simulink model "RajamaniController"  (R2018a)
settings: Solver=ode45  StartTime=0.0  StopTime=inf  FixedStep=0.002  RelTol=1e-3  EnableMultiTasking=on
values from neighbouring files (symbols this model uses):
  alpha_f0 = states(7)    [IS_2impulse.m]    (also in IS_3impulse.m; IS_4impulse.m; InputShaper.m; InputShaper2.m = 0)
  alpha_r0 = states(8)    [IS_2impulse.m]    (also in IS_3impulse.m; IS_4impulse.m; InputShaper.m; InputShaper2.m = 0)
  Bx_ash_f = 11.7    [ISData.m]    (also in SbWdata.m; pacjeka_params.m)
  Bx_ash_r = 11.1    [ISData.m]    (also in SbWdata.m; pacjeka_params.m)
  Bx_snow_f = 10.2    [ISData.m]    (also in SbWdata.m; pacjeka_params.m)
  Bx_snow_r = 9.71    [ISData.m]    (also in SbWdata.m; pacjeka_params.m)
  Bx_wash_f = 12    [ISData.m]    (also in SbWdata.m; pacjeka_params.m)
  Bx_wash_r = 11.5    [ISData.m]    (also in SbWdata.m; pacjeka_params.m)
  By_ash_f = 8.86    [ISData.m]    (also in SbWdata.m; pacjeka_params.m)
  By_ash_r = 9.30    (= 9.3)    [ISData.m]    (also in SbWdata.m; pacjeka_params.m)
  By_snow_f = 19.1    [ISData.m]    (also in SbWdata.m; pacjeka_params.m)
  By_snow_r = 20.0    (= 20)    [ISData.m]    (also in SbWdata.m; pacjeka_params.m)
  By_wash_f = 10.7    [ISData.m]    (also in SbWdata.m; pacjeka_params.m)
  By_wash_r = 11.3    [ISData.m]    (also in SbWdata.m; pacjeka_params.m)
  C_alpha_f = 1830*0.45*0.165*57.29578    (= 7785.20734695)    [IS_2impulse.m]    (also in IS_3impulse.m; IS_4impulse.m; InputShaper.m = 8650.2303855; InputShaper2.m = 8650.2303855)
  C_alpha_r = 1830*0.55*0.165*57.29578    (= 9515.25342405)    [IS_2impulse.m]    (also in IS_3impulse.m; IS_4impulse.m; InputShaper.m = 8650.2303855; InputShaper2.m = 8650.2303855)
  Cx_ash_f = 1.69    [ISData.m]    (also in SbWdata.m; pacjeka_params.m)
  Cx_ash_r = 1.69    [ISData.m]    (also in SbWdata.m; pacjeka_params.m)
  Cx_snow_f = 1.96    [ISData.m]    (also in SbWdata.m; pacjeka_params.m)
  Cx_snow_r = 1.96    [ISData.m]    (also in SbWdata.m; pacjeka_params.m)
  Cx_wash_f = 1.80    (= 1.8)    [ISData.m]    (also in SbWdata.m; pacjeka_params.m)
  Cx_wash_r = 1.80    (= 1.8)    [ISData.m]    (also in SbWdata.m; pacjeka_params.m)
  Cy_ash_f = 1.19    [ISData.m]    (also in SbWdata.m; pacjeka_params.m)
  Cy_ash_r = 1.19    [ISData.m]    (also in SbWdata.m; pacjeka_params.m)
  Cy_snow_f = 0.550    (= 0.55)    [ISData.m]    (also in SbWdata.m; pacjeka_params.m)
  Cy_snow_r = 0.550    (= 0.55)    [ISData.m]    (also in SbWdata.m; pacjeka_params.m)
  Cy_wash_f = 1.07    [ISData.m]    (also in SbWdata.m; pacjeka_params.m)
  Cy_wash_r = 1.07    [ISData.m]    (also in SbWdata.m; pacjeka_params.m)
  D_phi = 16000    [ISData.m]    (also in IS_2impulse.m; IS_3impulse.m; IS_4impulse.m; InputShaper.m)
  D_theta = 30960    [ISData.m]    (also in IS_2impulse.m; IS_3impulse.m; IS_4impulse.m; InputShaper.m)
  delta_r = 0    [ISData.m]    (also in IS_2impulse.m; IS_3impulse.m; IS_4impulse.m; InputShaper.m)
  epsilon = 0.4    [ISData.m]    (also in IS_2impulse.m; IS_3impulse.m; IS_4impulse.m; InputShaper.m)
  Ex_ash_f = 0.377    [ISData.m]    (also in SbWdata.m; pacjeka_params.m)
  Ex_ash_r = 0.362    [ISData.m]    (also in SbWdata.m; pacjeka_params.m)
  Ex_snow_f = 0.651    [ISData.m]    (also in SbWdata.m; pacjeka_params.m)
  Ex_snow_r = 0.624    [ISData.m]    (also in SbWdata.m; pacjeka_params.m)
  Ex_wash_f = 0.313    [ISData.m]    (also in SbWdata.m; pacjeka_params.m)
  Ex_wash_r = 0.300    (= 0.3)    [ISData.m]    (also in SbWdata.m; pacjeka_params.m)
  Ey_ash_f = -1.21    [ISData.m]    (also in SbWdata.m; pacjeka_params.m)
  Ey_ash_r = -1.11    [ISData.m]    (also in SbWdata.m; pacjeka_params.m)
  Ey_snow_f = -2.1    [ISData.m]    (also in SbWdata.m; pacjeka_params.m)
  Ey_snow_r = -1.93    [ISData.m]    (also in SbWdata.m; pacjeka_params.m)
  Ey_wash_f = -2.14    [ISData.m]    (also in SbWdata.m; pacjeka_params.m)
  Ey_wash_r = -1.97    [ISData.m]    (also in SbWdata.m; pacjeka_params.m)
  g = 9.81    [ISData.m]    (also in IS_2impulse.m; IS_3impulse.m; IS_4impulse.m; InputShaper.m)
  h = 0.5    [ISData.m]    (also in IS_2impulse.m; IS_3impulse.m; IS_4impulse.m; InputShaper.m)
  Iw = 4    [ISData.m]    (also in IS_2impulse.m; IS_3impulse.m; IS_4impulse.m; InputShaper.m)
  Ixx = 602.1923    [ISData.m]    (also in IS_2impulse.m; IS_3impulse.m; IS_4impulse.m; InputShaper.m)
  Iyy = 2.7370e+03    (= 2737)    [ISData.m]    (also in IS_2impulse.m; IS_3impulse.m; IS_4impulse.m; InputShaper.m)
  Iz = Izz    (= 3070)    [IS_2impulse.m]    (also in IS_3impulse.m; IS_4impulse.m; InputShaper.m; InputShaper2.m)
  Izz = 3070    [ISData.m]    (also in IS_2impulse.m; IS_3impulse.m; IS_4impulse.m; InputShaper.m)
  K_phi = 178000    [ISData.m]    (also in IS_2impulse.m; IS_3impulse.m; IS_4impulse.m; InputShaper.m)
  K_theta = 363540    [ISData.m]    (also in IS_2impulse.m; IS_3impulse.m; IS_4impulse.m; InputShaper.m)
  Ksbw = 1    [SbWdata.m]
  l = l_f+l_r    (= 2.67)    [IS_2impulse.m]    (also in IS_3impulse.m; IS_4impulse.m; InputShaper.m; InputShaper2.m)
  l_f = 1.2110    (= 1.211)    [ISData.m]    (also in IS_2impulse.m; IS_3impulse.m; IS_4impulse.m; InputShaper.m)
  l_p = Iz/(m*l_r)    (= 1.14982565347)    [IS_2impulse.m]    (also in IS_3impulse.m; IS_4impulse.m; InputShaper.m; InputShaper2.m)
  l_r = 1.4590    (= 1.459)    [ISData.m]    (also in IS_2impulse.m; IS_3impulse.m; IS_4impulse.m; InputShaper.m)
  m = 1830    [ISData.m]    (also in IS_2impulse.m; IS_3impulse.m; IS_4impulse.m; InputShaper.m)
  mu_x_ash_f = 1.20    (= 1.2)    [ISData.m]    (also in SbWdata.m; pacjeka_params.m)
  mu_x_ash_r = 1.20    (= 1.2)    [ISData.m]    (also in SbWdata.m; pacjeka_params.m)
  mu_x_snow_f = 0.407    [ISData.m]    (also in SbWdata.m; pacjeka_params.m)
  mu_x_snow_r = 0.409    [ISData.m]    (also in SbWdata.m; pacjeka_params.m)
  mu_x_wash_f = 1.06    [ISData.m]    (also in SbWdata.m; pacjeka_params.m)
  mu_x_wash_r = 1.07    [ISData.m]    (also in SbWdata.m; pacjeka_params.m)
  mu_y_ash_f = 0.935    [ISData.m]    (also in SbWdata.m; pacjeka_params.m)
  mu_y_ash_r = 0.961    [ISData.m]    (also in SbWdata.m; pacjeka_params.m)
  mu_y_snow_f = 0.383    [ISData.m]    (also in SbWdata.m; pacjeka_params.m)
  mu_y_snow_r = 0.394    [ISData.m]    (also in SbWdata.m; pacjeka_params.m)
  mu_y_wash_f = 0.885    [ISData.m]    (also in SbWdata.m; pacjeka_params.m)
  mu_y_wash_r = 0.911    [ISData.m]    (also in SbWdata.m; pacjeka_params.m)
  omega0 = Vx0/Rw    (= 64.7813411079)    [ISData.m]    (also in IS_2impulse.m = 74.1; IS_3impulse.m = 74.1; IS_4impulse.m = 74.1; InputShaper.m = 55.5666666667)
  omega_f0 = states(5)    [IS_2impulse.m]    (also in IS_3impulse.m; IS_4impulse.m; InputShaper.m; InputShaper2.m = 55.5666666667)
  omega_r0 = states(6)    [IS_2impulse.m]    (also in IS_3impulse.m; IS_4impulse.m; InputShaper.m; InputShaper2.m = 55.5666666667)
  psi0 = states(2)    [IS_2impulse.m]    (also in IS_3impulse.m; IS_4impulse.m; InputShaper.m; InputShaper2.m = 0)
  psi_dot0 = states(1)    [IS_2impulse.m]    (also in IS_3impulse.m; IS_4impulse.m; InputShaper.m; InputShaper2.m = 0)
  Px0 = states(9)    [IS_2impulse.m]    (also in IS_3impulse.m; IS_4impulse.m; InputShaper.m; InputShaper2.m = 0)
  Py0 = states(10)    [IS_2impulse.m]    (also in IS_3impulse.m; IS_4impulse.m; InputShaper.m; InputShaper2.m = 0)
  Re = Rw    (= 0.3)    [IS_2impulse.m]    (also in IS_3impulse.m; IS_4impulse.m; InputShaper.m; InputShaper2.m)
  road = 1    [ISData.m]    (also in IS_2impulse.m; IS_3impulse.m; IS_4impulse.m; InputShaper.m)
  Rw = 0.3430    (= 0.343)    [ISData.m]    (also in IS_2impulse.m = 0.3; IS_3impulse.m = 0.3; IS_4impulse.m = 0.3; InputShaper.m = 0.3)
  sigma = epsilon    (= 0.4)    [IS_2impulse.m]    (also in IS_3impulse.m; IS_4impulse.m; InputShaper.m; InputShaper2.m)
  Ts = 0.001    [ISData.m]    (also in IS_2impulse.m; IS_3impulse.m; IS_4impulse.m; InputShaper.m)
  Tsmall = 0.001    [ISData.m]    (also in IS_2impulse.m; IS_3impulse.m; IS_4impulse.m; InputShaper.m)
  Vx0 = 22.22    [ISData.m]    (also in IS_2impulse.m = states(3); IS_3impulse.m = states(3); IS_4impulse.m = states(3); InputShaper.m = states(3))
  Vy0 = states(4)    [IS_2impulse.m]    (also in IS_3impulse.m; IS_4impulse.m; InputShaper.m; InputShaper2.m = 0)
  w = 0.7700    (= 0.77)    [ISData.m]    (also in IS_2impulse.m; IS_3impulse.m; IS_4impulse.m; InputShaper.m)
(part 3 of 3)

== system RajamaniController/Vehicle_Sim/Vehicle_model/phi_subsystem/phi_ddot_numerator_subsystem ==
  FY : Inport  OutDataTypeStr=double  SampleTime=Ts
  psi_dot : Inport  Port=2  OutDataTypeStr=double  SampleTime=Tsmall
  phi_dot : Inport  Port=3  OutDataTypeStr=double  SampleTime=Tsmall
  phi : Inport  Port=4  OutDataTypeStr=double  SampleTime=Tsmall
  theta_dot : Inport  Port=5  OutDataTypeStr=double  SampleTime=Tsmall
  theta : Inport  Port=6  OutDataTypeStr=double  SampleTime=Tsmall
  Iyy : Inport  Port=7  OutDataTypeStr=double  SampleTime=Ts
  Izz : Inport  Port=8  OutDataTypeStr=double  SampleTime=Ts
  K_phi : Inport  Port=9  OutDataTypeStr=double  SampleTime=Ts
  D_phi : Inport  Port=10  OutDataTypeStr=double  SampleTime=Ts
  h : Inport  Port=11  OutDataTypeStr=double  SampleTime=Ts
  Add : Sum
  Add1 : Sum  Inputs=+++
  Add2 : Sum
  Add3 : Sum  Inputs=+-
  Add4 : Sum
  Add7 : Sum  Inputs=+++
  Divide{,1..4,7..12} (11 alike) : Product  Inputs=**
  Divide5 : Product  Inputs=****
  Divide6 : Product  Inputs=****
  Gain : Gain  Gain=m*g
  Gain2 : Gain  Gain=-1
  Gain3 : Gain  Gain=-1
  Square : Math  Operator=square  RndMeth=Zero  SaturateOnIntegerOverflow=on
  Square1 : Math  Operator=square  RndMeth=Zero  SaturateOnIntegerOverflow=on
  Trigonometric Function : Trigonometry
  Trigonometric Function1 : Trigonometry  Operator=cos
  Trigonometric Function2 : Trigonometry  Operator=cos
  Trigonometric Function3 : Trigonometry
  phi_ddot_numerator : Outport  OutDataTypeStr=double  SampleTime=Tsmall
  wires:
  phi_dot/1 -> Divide1/1, Divide6/3  "phi_dot"
  psi_dot/1 -> Divide4/1, Divide5/4, Divide11/2  "psi_dot"
  Divide6/1 -> Add4/2
  phi/1 -> Divide/1, Trigonometric Function/1, Trigonometric Function1/1  "phi"
  theta/1 -> Trigonometric Function2/1, Trigonometric Function3/1  "theta"
  FY/1 -> Divide2/1  "FY"
  theta_dot/1 -> Divide11/1  "theta_dot"
  Gain2/1 -> Divide/2
  Gain3/1 -> Divide1/2
  Divide1/1 -> Add1/2
  Divide9/1 -> Add2/2
  Divide12/1 -> Add1/3
  Add/1 -> Divide12/1
  Divide3/1 -> Add/2
  Add2/1 -> Divide10/1
  Iyy/1 -> Divide9/2, Add3/1  "Iyy"
  Divide2/1 -> Divide3/1
  Square1/1 -> Divide8/2
  Izz/1 -> Add3/2, Divide8/1  "Izz"
  Add3/1 -> Divide4/2  "del_Iyz"
  Gain/1 -> Add/1
  Add7/1 -> phi_ddot_numerator/1
  Divide8/1 -> Add2/1
  Divide4/1 -> Divide7/1
  Add4/1 -> Divide7/2
  Trigonometric Function2/1 -> Divide3/2, Divide5/3  "cosTheta"
  Divide11/1 -> Divide10/2
  Divide5/1 -> Add4/1
  Divide7/1 -> Add7/2
  Square/1 -> Divide9/1
  Trigonometric Function1/1 -> Divide2/2, Divide5/2, Square/1, Divide6/2  "cosPhi"
  Divide10/1 -> Add7/3
  Add1/1 -> Add7/1
  Trigonometric Function3/1 -> Divide6/4  "sinTheta"
  Divide/1 -> Add1/1
  Trigonometric Function/1 -> Divide5/1, Divide6/1, Square1/1, Gain/1  "sinPhi"
  K_phi/1 -> Gain2/1  "K_phi"
  D_phi/1 -> Gain3/1  "D_phi"
  h/1 -> Divide12/2  "h"

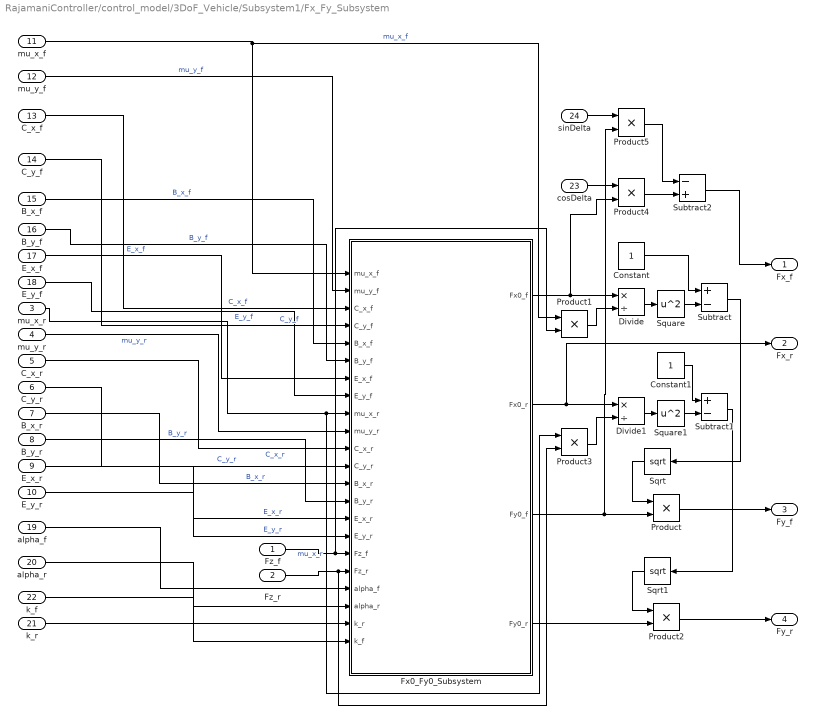
== system RajamaniController/control_model/3DoF_Vehicle/Subsystem1/Fx_Fy_Subsystem ==
  Fz_f : Inport
  Fz_r : Inport  Port=2
  mu_x_r : Inport  Port=3
  mu_y_r : Inport  Port=4
  C_x_r : Inport  Port=5
  C_y_r : Inport  Port=6
  B_x_r : Inport  Port=7
  B_y_r : Inport  Port=8
  E_x_r : Inport  Port=9
  E_y_r : Inport  Port=10
  mu_x_f : Inport  Port=11
  mu_y_f : Inport  Port=12
  C_x_f : Inport  Port=13
  C_y_f : Inport  Port=14
  B_x_f : Inport  Port=15
  B_y_f : Inport  Port=16
  E_x_f : Inport  Port=17
  E_y_f : Inport  Port=18
  alpha_f : Inport  Port=19
  alpha_r : Inport  Port=20
  k_r : Inport  Port=21
  k_f : Inport  Port=22
  cosDelta : Inport  Port=23
  sinDelta : Inport  Port=24
  Constant : Constant
  Constant1 : Constant
  Divide : Product  Inputs=*/
  Divide1 : Product  Inputs=*/
  Fx0_Fy0_Subsystem : Subsystem
  Product{,1..5} (6 alike) : Product
  Sqrt : Sqrt  SaturateOnIntegerOverflow=on
  Sqrt1 : Sqrt  SaturateOnIntegerOverflow=on
  Square : Math  Operator=square  SaturateOnIntegerOverflow=on
  Square1 : Math  Operator=square  SaturateOnIntegerOverflow=on
  Subtract : Sum  Inputs=+-
  Subtract1 : Sum  Inputs=+-
  Subtract2 : Sum  Inputs=-+
  Fx_f : Outport
  Fx_r : Outport  Port=2
  Fy_f : Outport  Port=3
  Fy_r : Outport  Port=4
  wires:
  B_x_r/1 -> Fx0_Fy0_Subsystem/13(B_x_r)  "B_x_r"
  mu_y_r/1 -> Fx0_Fy0_Subsystem/10(mu_y_r)  "mu_y_r"
  C_x_r/1 -> Fx0_Fy0_Subsystem/11(C_x_r)  "C_x_r"
  E_y_r/1 -> Fx0_Fy0_Subsystem/16(E_y_r)  "E_y_r"
  mu_x_r/1 -> Fx0_Fy0_Subsystem/9(mu_x_r), Product3/1  "mu_x_r"
  C_y_r/1 -> Fx0_Fy0_Subsystem/12(C_y_r)  "C_y_r"
  E_x_r/1 -> Fx0_Fy0_Subsystem/15(E_x_r)  "E_x_r"
  B_y_r/1 -> Fx0_Fy0_Subsystem/14(B_y_r)  "B_y_r"
  B_x_f/1 -> Fx0_Fy0_Subsystem/5(B_x_f)  "B_x_f"
  mu_y_f/1 -> Fx0_Fy0_Subsystem/2(mu_y_f)  "mu_y_f"
  C_x_f/1 -> Fx0_Fy0_Subsystem/3(C_x_f)  "C_x_f"
  E_y_f/1 -> Fx0_Fy0_Subsystem/8(E_y_f)  "E_y_f"
  mu_x_f/1 -> Product1/1, Fx0_Fy0_Subsystem/1(mu_x_f)  "mu_x_f"
  C_y_f/1 -> Fx0_Fy0_Subsystem/4(C_y_f)  "C_y_f"
  E_x_f/1 -> Fx0_Fy0_Subsystem/7(E_x_f)  "E_x_f"
  B_y_f/1 -> Fx0_Fy0_Subsystem/6(B_y_f)  "B_y_f"
  Fz_f/1 -> Product1/2, Fx0_Fy0_Subsystem/17(Fz_f)
  Fz_r/1 -> Product3/2, Fx0_Fy0_Subsystem/18(Fz_r)
  alpha_f/1 -> Fx0_Fy0_Subsystem/19(alpha_f)
  alpha_r/1 -> Fx0_Fy0_Subsystem/20(alpha_r)
  k_f/1 -> Fx0_Fy0_Subsystem/22(k_f)
  k_r/1 -> Fx0_Fy0_Subsystem/21(k_r)
  Constant/1 -> Subtract/1
  Fx0_Fy0_Subsystem/1(Fx0_f) -> Product4/2, Divide/1
  Product1/1 -> Divide/2
  Divide/1 -> Square/1
  Subtract/1 -> Sqrt/1
  Square/1 -> Subtract/2
  Sqrt/1 -> Product/1
  Product/1 -> Fy_f/1
  Product2/1 -> Fy_r/1
  Fx0_Fy0_Subsystem/4(Fy0_r) -> Product2/2
  Sqrt1/1 -> Product2/1
  Divide1/1 -> Square1/1
  Square1/1 -> Subtract1/2
  Product3/1 -> Divide1/2
  Fx0_Fy0_Subsystem/2(Fx0_r) -> Fx_r/1, Divide1/1
  Constant1/1 -> Subtract1/1
  Subtract1/1 -> Sqrt1/1
  cosDelta/1 -> Product4/1
  Product4/1 -> Subtract2/2
  sinDelta/1 -> Product5/1
  Fx0_Fy0_Subsystem/3(Fy0_f) -> Product5/2, Product/2
  Product5/1 -> Subtract2/1
  Subtract2/1 -> Fx_f/1

== system RajamaniController/control_model/3DoF_Vehicle/Subsystem1/Fz_Subsystem ==
  Constant : Constant  Value=(m*g*l_f)/l
  Constant1 : Constant  Value=(m*g*l_r)/l
  Fz_f : Outport
  Fz_r : Outport  Port=2
  wires:
  Constant/1 -> Fz_r/1
  Constant1/1 -> Fz_f/1

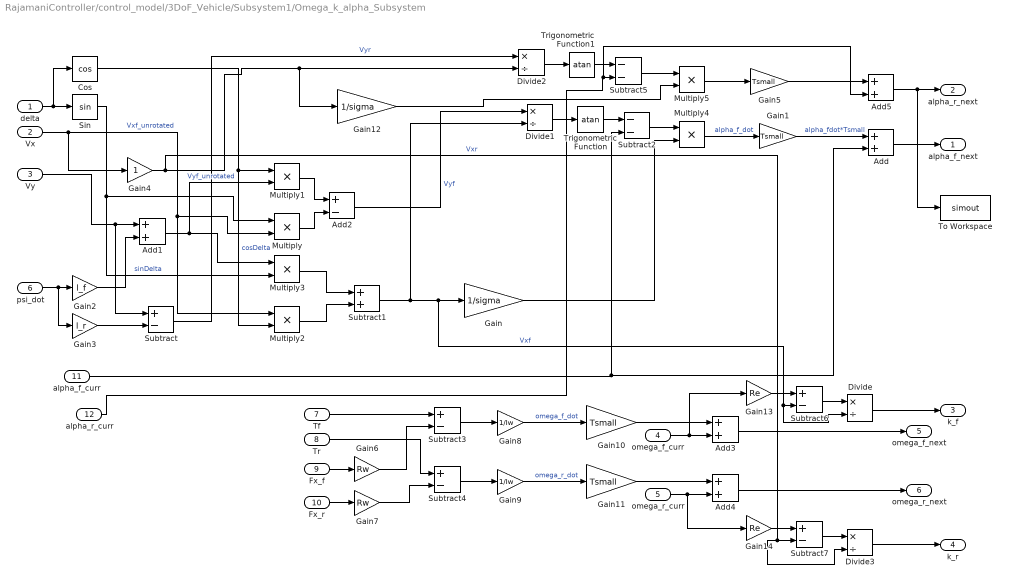
== system RajamaniController/control_model/3DoF_Vehicle/Subsystem1/Omega_k_alpha_Subsystem ==
  delta : Inport
  Vx : Inport  Port=2
  Vy : Inport  Port=3
  omega_f_curr : Inport  Port=4
  omega_r_curr : Inport  Port=5
  psi_dot : Inport  Port=6
  Tf : Inport  Port=7
  Tr : Inport  Port=8
  Fx_f : Inport  Port=9
  Fx_r : Inport  Port=10
  alpha_f_curr : Inport  Port=11
  alpha_r_curr : Inport  Port=12
  Add{,1,3..5} (5 alike) : Sum
  Add2 : Sum  Inputs=+-
  Cos : Trigonometry  Operator=cos
  Divide{,1..3} (4 alike) : Product  Inputs=*/
  Gain : Gain  Gain=1/sigma
  Gain{1,5,10..11} (4 alike) : Gain  Gain=Tsmall
  Gain12 : Gain  Gain=1/sigma
  Gain13 : Gain  Gain=Re
  Gain14 : Gain  Gain=Re
  Gain2 : Gain  Gain=l_f
  Gain3 : Gain  Gain=l_r
  Gain4 : Gain
  Gain6 : Gain  Gain=Rw
  Gain7 : Gain  Gain=Rw
  Gain8 : Gain  Gain=1/Iw
  Gain9 : Gain  Gain=1/Iw
  Multiply{,1..5} (6 alike) : Product
  Sin : Trigonometry
  Subtract{,3..4,6..7} (5 alike) : Sum  Inputs=+-
  Subtract1 : Sum
  Subtract2 : Sum  Inputs=--
  Subtract5 : Sum  Inputs=--
  To Workspace : ToWorkspace  VariableName=simout  SaveFormat=Timeseries  SampleTime=-1
  Trigonometric Function : Trigonometry  Operator=atan
  Trigonometric Function1 : Trigonometry  Operator=atan
  alpha_f_next : Outport
  alpha_r_next : Outport  Port=2
  k_f : Outport  Port=3
  k_r : Outport  Port=4
  omega_f_next : Outport  Port=5
  omega_r_next : Outport  Port=6
  wires:
  Fx_f/1 -> Gain6/1
  Fx_r/1 -> Gain7/1
  Tf/1 -> Subtract3/1
  Gain6/1 -> Subtract3/2
  Tr/1 -> Subtract4/1
  Gain7/1 -> Subtract4/2
  Subtract3/1 -> Gain8/1
  Subtract4/1 -> Gain9/1
  Gain8/1 -> Gain10/1  "omega_f_dot"
  Gain9/1 -> Gain11/1  "omega_r_dot"
  Gain10/1 -> Add3/1
  Gain11/1 -> Add4/1
  Add3/1 -> omega_f_next/1
  Add4/1 -> omega_r_next/1
  omega_f_curr/1 -> Gain13/1, Add3/2
  Multiply4/1 -> Gain1/1  "alpha_f_dot"
  Gain1/1 -> Add/1  "alpha_fdot*Tsmall"
  Divide1/1 -> Trigonometric Function/1
  omega_r_curr/1 -> Gain14/1, Add4/2
  psi_dot/1 -> Gain3/1, Gain2/1
  Gain2/1 -> Add1/2
  Vy/1 -> Subtract/1, Add1/1
  Add1/1 -> Multiply1/2, Multiply3/1  "Vyf_unrotated"
  Gain3/1 -> Subtract/2
  Subtract/1 -> Divide2/1  "Vyr"
  Vx/1 -> Multiply/2, Multiply2/1, Gain4/1  "Vxf_unrotated"
  Gain4/1 -> Subtract7/2, Divide3/2, Gain12/1, Divide2/2  "Vxr"
  delta/1 -> Cos/1, Sin/1
  Cos/1 -> Multiply2/2, Multiply1/1  "cosDelta"
  Multiply1/1 -> Add2/1
  Multiply/1 -> Add2/2
  Add2/1 -> Divide1/1  "Vyf"
  Multiply3/1 -> Subtract1/1
  Multiply2/1 -> Subtract1/2
  Subtract1/1 -> Divide/2, Subtract6/2, Gain/1, Divide1/2  "Vxf"
  Trigonometric Function/1 -> Subtract2/1
  alpha_f_curr/1 -> Add/2, Subtract2/2
  Subtract2/1 -> Multiply4/1
  Gain/1 -> Multiply4/2
  Add/1 -> alpha_f_next/1
  Subtract5/1 -> Multiply5/1
  Trigonometric Function1/1 -> Subtract5/1
  Divide2/1 -> Trigonometric Function1/1
  Multiply5/1 -> Gain5/1
  Gain5/1 -> Add5/1
  Add5/1 -> To Workspace/1, alpha_r_next/1
  alpha_r_curr/1 -> Add5/2, Subtract5/2
  Gain12/1 -> Multiply5/2
  Gain13/1 -> Subtract6/1
  Subtract6/1 -> Divide/1
  Divide/1 -> k_f/1
  Gain14/1 -> Subtract7/1
  Subtract7/1 -> Divide3/1
  Divide3/1 -> k_r/1
  Sin/1 -> Multiply/1, Multiply3/2  "sinDelta"

== system RajamaniController/control_model/3DoF_Vehicle/Subsystem1/Pacjeka_parameters_Subsystem ==
  surface_condition : Inport  OutDataTypeStr=double  SampleTime=Ts
  Ashphalt_condition_subsystem : Subsystem  TreatAsAtomicUnit=on
  Demux : Demux  Outputs=2
  Ice_condition_subsystem : Subsystem  TreatAsAtomicUnit=on
  Merge : Merge  Inputs=4
  Snow_condition_subsystem : Subsystem  TreatAsAtomicUnit=on
  Switch Case : SwitchCase  CaseConditions={1,2,3,4}  ShowDefaultCase=off
  WetAshphalt_condition_subsystem : Subsystem  TreatAsAtomicUnit=on
  front : Outport  OutDataTypeStr=double  SampleTime=Ts
  rear : Outport  Port=2  OutDataTypeStr=double  SampleTime=Ts
  wires:
  Demux/2 -> rear/1  "rear"
  Merge/1 -> Demux/1
  Switch Case/1 -> Ashphalt_condition_subsystem/Action
  Switch Case/3 -> Snow_condition_subsystem/Action
  Demux/1 -> front/1  "front"
  surface_condition/1 -> Switch Case/1
  Ashphalt_condition_subsystem/1(Out1) -> Merge/1
  Switch Case/2 -> WetAshphalt_condition_subsystem/Action
  WetAshphalt_condition_subsystem/1(Out1) -> Merge/2
  Snow_condition_subsystem/1(Out1) -> Merge/3
  Ice_condition_subsystem/1(Out1) -> Merge/4
  Switch Case/4 -> Ice_condition_subsystem/Action

== system RajamaniController/control_model/3DoF_Vehicle/Subsystem1/Psi_ddot_subsystem ==
  cosDelta : Inport
  sinDelta : Inport  Port=2
  Fyf : Inport  Port=3
  Fyr : Inport  Port=4
  Fxf : Inport  Port=5
  psi_dot_curr : Inport  Port=6
  Add : Sum  Inputs=++-
  Add1 : Sum
  Gain : Gain  Gain=l_f
  Gain1 : Gain  Gain=l_r
  Gain2 : Gain  Gain=l_f
  Gain3 : Gain  Gain=1/Iz
  Gain4 : Gain  Gain=Tsmall
  Multiply : Product
  Multiply1 : Product
  psi_dot_next : Outport
  psi_ddot : Outport  Port=2
  wires:
  cosDelta/1 -> Multiply/1
  Fyf/1 -> Multiply/2
  Multiply/1 -> Gain/1
  Fyr/1 -> Gain1/1
  sinDelta/1 -> Multiply1/1
  Fxf/1 -> Multiply1/2
  Multiply1/1 -> Gain2/1
  Gain/1 -> Add/1
  Gain2/1 -> Add/2
  Gain1/1 -> Add/3
  Add/1 -> Gain3/1  "Mz"
  Gain3/1 -> psi_ddot/1, Gain4/1  "psi_ddot"
  Gain4/1 -> Add1/1
  psi_dot_curr/1 -> Add1/2
  Add1/1 -> psi_dot_next/1  "psi_dot_next"

== system RajamaniController/control_model/3DoF_Vehicle/Subsystem1/Vxdot_subsystem ==
  psi_dot_curr : Inport
  Vy_curr : Inport  Port=2
  Fxf : Inport  Port=3
  Fxr : Inport  Port=4
  Fyf : Inport  Port=5
  cosDelta : Inport  Port=6
  sinDelta : Inport  Port=7
  Vx_curr : Inport  Port=8
  Add : Sum
  Fy_subsystem : Subsystem
  Gain : Gain  Gain=1/m
  Gain1 : Gain  Gain=Ts
  Multiply : Product
  Subtract : Sum
  Vx_next : Outport
  Ax : Outport  Port=2
  wires:
  sinDelta/1 -> Fy_subsystem/5(sinDelta)
  cosDelta/1 -> Fy_subsystem/4(cosDelta)
  Fyf/1 -> Fy_subsystem/3(Fxr)
  Fxr/1 -> Fy_subsystem/2(Fxf)
  Fxf/1 -> Fy_subsystem/1(Fyf)
  Fy_subsystem/1(Fx) -> Gain/1
  Gain/1 -> Subtract/2
  psi_dot_curr/1 -> Multiply/1
  Vy_curr/1 -> Multiply/2
  Multiply/1 -> Subtract/1
  Subtract/1 -> Ax/1, Gain1/1
  Gain1/1 -> Add/1
  Vx_curr/1 -> Add/2
  Add/1 -> Vx_next/1  "Vx_next"

== system RajamaniController/control_model/3DoF_Vehicle/Subsystem1/Vydot_subsystem ==
  psi_dot_curr : Inport
  Vx_curr : Inport  Port=2
  Fyf : Inport  Port=3
  Fyr : Inport  Port=4
  Fxf : Inport  Port=5
  cosDelta : Inport  Port=6
  sinDelta : Inport  Port=7
  Vy_curr : Inport  Port=8
  Add : Sum
  Fy_subsystem : Subsystem
  Gain : Gain  Gain=1/m
  Gain1 : Gain  Gain=Ts
  Multiply : Product
  Subtract : Sum  Inputs=-+
  Vy_next : Outport
  wires:
  sinDelta/1 -> Fy_subsystem/5(sinDelta)
  cosDelta/1 -> Fy_subsystem/4(cosDelta)
  Fxf/1 -> Fy_subsystem/3(Fxf)
  Fyr/1 -> Fy_subsystem/2(Fyr)
  Fyf/1 -> Fy_subsystem/1(Fyf)
  Fy_subsystem/1(Fy) -> Gain/1
  Gain/1 -> Subtract/2
  psi_dot_curr/1 -> Multiply/1
  Vx_curr/1 -> Multiply/2
  Multiply/1 -> Subtract/1
  Subtract/1 -> Gain1/1
  Gain1/1 -> Add/1
  Vy_curr/1 -> Add/2
  Add/1 -> Vy_next/1  "Vy_next"

== system RajamaniController/Vehicle_Sim/Vehicle_model/omega_alpha_and_k_values_subsystem/Subsystem5/Subsystem ==
  Vx1_ur : Inport
  Vy1_ur : Inport  Port=2
  cosDeltaf2 : Inport  Port=3
  sinDeltaf2 : Inport  Port=4
  Add3 : Sum
  Multiply{3..6} (4 alike) : Product
  Subtract1 : Sum  Inputs=+-
  Vx1 : Outport
  Vy1 : Outport  Port=2
  wires:
  Subtract1/1 -> Vy1/1  "Vy1"
  Multiply6/1 -> Add3/2
  Multiply5/1 -> Add3/1
  sinDeltaf2/1 -> Multiply4/2, Multiply6/2
  cosDeltaf2/1 -> Multiply3/2, Multiply5/2
  Vx1_ur/1 -> Multiply4/1, Multiply5/1
  Multiply3/1 -> Subtract1/1
  Vy1_ur/1 -> Multiply3/1, Multiply6/1
  Multiply4/1 -> Subtract1/2
  Add3/1 -> Vx1/1  "Vx1"

== system RajamaniController/Vehicle_Sim/Vehicle_model/omega_alpha_and_k_values_subsystem/Subsystem5/Subsystem1 ==
  Vx2_ur : Inport
  Vy2_ur : Inport  Port=2
  cosDeltaf2 : Inport  Port=3
  sinDeltaf2 : Inport  Port=4
  Add4 : Sum
  Multiply{7..10} (4 alike) : Product
  Subtract2 : Sum  Inputs=+-
  Vx2 : Outport
  Vy2 : Outport  Port=2
  wires:
  Vx2_ur/1 -> Multiply9/2, Multiply8/2
  sinDeltaf2/1 -> Multiply8/1, Multiply10/1
  Vy2_ur/1 -> Multiply10/2, Multiply7/2
  Add4/1 -> Vx2/1  "Vx2"
  Multiply10/1 -> Add4/2
  cosDeltaf2/1 -> Multiply7/1, Multiply9/1
  Multiply9/1 -> Add4/1
  Multiply8/1 -> Subtract2/2
  Multiply7/1 -> Subtract2/1
  Subtract2/1 -> Vy2/1  "Vy2"

== system RajamaniController/Vehicle_Sim/Vehicle_model/omega_alpha_and_k_values_subsystem/Subsystem5/Subsystem2 ==
  cosDelta_r : Inport
  sinDelta_r : Inport  Port=2
  Vx3_ur : Inport  Port=3
  Vy3_ur : Inport  Port=4
  Add3 : Sum
  Multiply{3..6} (4 alike) : Product
  Subtract1 : Sum  Inputs=+-
  Vx3 : Outport
  Vy3 : Outport  Port=2
  wires:
  Vy3_ur/1 -> Multiply3/1, Multiply6/2
  sinDelta_r/1 -> Multiply4/1, Multiply6/1
  Multiply3/1 -> Subtract1/1
  Multiply6/1 -> Add3/2
  Multiply4/1 -> Subtract1/2
  Multiply5/1 -> Add3/1
  Vx3_ur/1 -> Multiply4/2, Multiply5/2
  Add3/1 -> Vx3/1  "Vx3"
  cosDelta_r/1 -> Multiply3/2, Multiply5/1
  Subtract1/1 -> Vy3/1  "Vy3"

== system RajamaniController/Vehicle_Sim/Vehicle_model/omega_alpha_and_k_values_subsystem/Subsystem5/Subsystem3 ==
  cosDelta_r : Inport
  sinDelta_r : Inport  Port=2
  Vx4_ur : Inport  Port=3
  Vy4_ur : Inport  Port=4
  Add3 : Sum
  Multiply{3..6} (4 alike) : Product
  Subtract1 : Sum  Inputs=+-
  Vx4 : Outport
  Vy4 : Outport  Port=2
  wires:
  Multiply6/1 -> Add3/2
  Multiply5/1 -> Add3/1
  sinDelta_r/1 -> Multiply4/1, Multiply6/1
  Vy4_ur/1 -> Multiply6/2, Multiply3/2
  Add3/1 -> Vx4/1  "Vx4"
  Multiply4/1 -> Subtract1/2
  Multiply3/1 -> Subtract1/1
  Subtract1/1 -> Vy4/1  "Vy4"
  cosDelta_r/1 -> Multiply5/1, Multiply3/1
  Vx4_ur/1 -> Multiply4/2, Multiply5/2

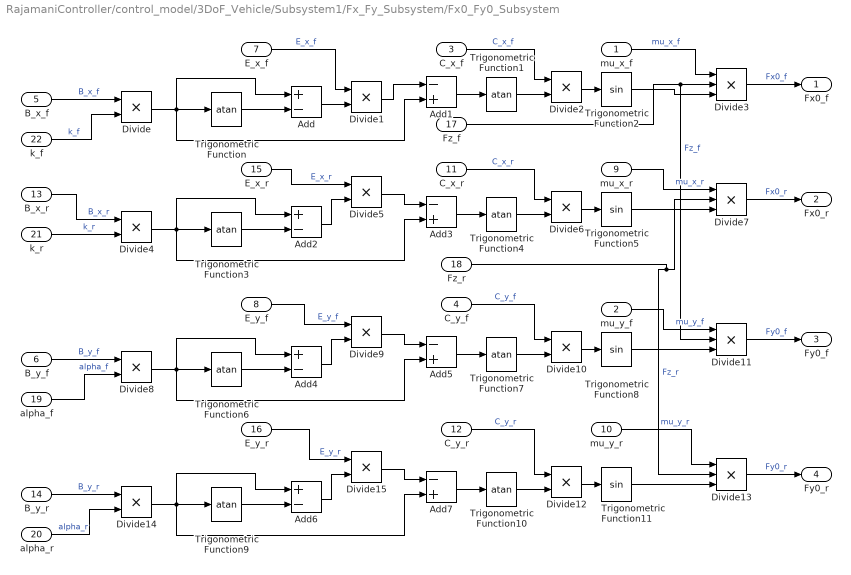
== system RajamaniController/control_model/3DoF_Vehicle/Subsystem1/Fx_Fy_Subsystem/Fx0_Fy0_Subsystem ==
  mu_x_f : Inport
  mu_y_f : Inport  Port=2
  C_x_f : Inport  Port=3
  C_y_f : Inport  Port=4
  B_x_f : Inport  Port=5
  B_y_f : Inport  Port=6
  E_x_f : Inport  Port=7
  E_y_f : Inport  Port=8
  mu_x_r : Inport  Port=9
  mu_y_r : Inport  Port=10
  C_x_r : Inport  Port=11
  C_y_r : Inport  Port=12
  B_x_r : Inport  Port=13
  B_y_r : Inport  Port=14
  E_x_r : Inport  Port=15
  E_y_r : Inport  Port=16
  Fz_f : Inport  Port=17
  Fz_r : Inport  Port=18
  alpha_f : Inport  Port=19
  alpha_r : Inport  Port=20
  k_r : Inport  Port=21
  k_f : Inport  Port=22
  Add{,2,4,6} (4 alike) : Sum  Inputs=+-
  Add{1,3,5,7} (4 alike) : Sum  Inputs=-+
  Divide{,1..2,4..6,8..10,12,14..15} (12 alike) : Product  Inputs=**
  Divide{3,7,11,13} (4 alike) : Product  Inputs=***
  Trigonometric Function{,1,3..4,6..7,9..10} (8 alike) : Trigonometry  Operator=atan
  Trigonometric Function{2,5,8,11} (4 alike) : Trigonometry
  Fx0_f : Outport
  Fx0_r : Outport  Port=2
  Fy0_f : Outport  Port=3
  Fy0_r : Outport  Port=4
  wires:
  E_y_f/1 -> Divide9/1  "E_y_f"
  B_x_f/1 -> Divide/1  "B_x_f"
  C_x_f/1 -> Divide2/1  "C_x_f"
  mu_x_f/1 -> Divide3/1  "mu_x_f"
  mu_y_f/1 -> Divide11/1  "mu_y_f"
  E_x_f/1 -> Divide1/1  "E_x_f"
  B_y_f/1 -> Divide8/1  "B_y_f"
  C_y_f/1 -> Divide10/1  "C_y_f"
  B_y_r/1 -> Divide14/1  "B_y_r"
  E_x_r/1 -> Divide5/1  "E_x_r"
  mu_x_r/1 -> Divide7/1  "mu_x_r"
  E_y_r/1 -> Divide15/1  "E_y_r"
  B_x_r/1 -> Divide4/1  "B_x_r"
  mu_y_r/1 -> Divide13/1  "mu_y_r"
  C_y_r/1 -> Divide12/1  "C_y_r"
  C_x_r/1 -> Divide6/1  "C_x_r"
  Trigonometric Function2/1 -> Divide3/3
  Divide3/1 -> Fx0_f/1  "Fx0_f"
  Divide5/1 -> Add3/1
  Trigonometric Function5/1 -> Divide7/3
  Add3/1 -> Trigonometric Function4/1
  Divide2/1 -> Trigonometric Function2/1
  Add1/1 -> Trigonometric Function1/1
  Trigonometric Function4/1 -> Divide6/2
  Divide7/1 -> Fx0_r/1  "Fx0_r"
  Add/1 -> Divide1/2
  Divide6/1 -> Trigonometric Function5/1
  Trigonometric Function3/1 -> Add2/2
  Divide/1 -> Add1/2, Add/1, Trigonometric Function/1
  Divide4/1 -> Add3/2, Add2/1, Trigonometric Function3/1
  Trigonometric Function1/1 -> Divide2/2
  Divide1/1 -> Add1/1
  Trigonometric Function/1 -> Add/2
  Add2/1 -> Divide5/2
  alpha_f/1 -> Divide8/2  "alpha_f"
  alpha_r/1 -> Divide14/2  "alpha_r"
  k_f/1 -> Divide/2  "k_f"
  k_r/1 -> Divide4/2  "k_r"
  Add4/1 -> Divide9/2
  Trigonometric Function7/1 -> Divide10/2
  Trigonometric Function6/1 -> Add4/2
  Divide10/1 -> Trigonometric Function8/1
  Divide9/1 -> Add5/1
  Fz_f/1 -> Divide11/2, Divide3/2  "Fz_f"
  Divide8/1 -> Add5/2, Add4/1, Trigonometric Function6/1
  Add5/1 -> Trigonometric Function7/1
  Trigonometric Function8/1 -> Divide11/3
  Divide11/1 -> Fy0_f/1  "Fy0_f"
  Divide13/1 -> Fy0_r/1  "Fy0_r"
  Divide14/1 -> Trigonometric Function9/1, Add7/2, Add6/1
  Fz_r/1 -> Divide13/2, Divide7/2  "Fz_r"
  Add7/1 -> Trigonometric Function10/1
  Add6/1 -> Divide15/2
  Trigonometric Function10/1 -> Divide12/2
  Divide15/1 -> Add7/1
  Trigonometric Function9/1 -> Add6/2
  Trigonometric Function11/1 -> Divide13/3
  Divide12/1 -> Trigonometric Function11/1

== system RajamaniController/control_model/3DoF_Vehicle/Subsystem1/Pacjeka_parameters_Subsystem/Ashphalt_condition_subsystem ==
  Action Port : ActionPort  ActionType=case
  Bx_ash_f : Constant  Value=Bx_ash_f
  Bx_ash_r : Constant  Value=Bx_ash_r
  By_ash_f : Constant  Value=By_ash_f
  By_ash_r : Constant  Value=By_ash_r
  Cx_ash_f : Constant  Value=Cx_ash_f
  Cx_ash_r : Constant  Value=Cx_ash_r
  Cy_ash_f : Constant  Value=Cy_ash_f
  Cy_ash_r : Constant  Value=Cy_ash_r
  Ex_ash_f : Constant  Value=Ex_ash_f
  Ex_ash_r : Constant  Value=Ex_ash_r
  Ey_ash_f : Constant  Value=Ey_ash_f
  Ey_ash_r : Constant  Value=Ey_ash_r
  Mux : Mux  Inputs=16
      settings: DisplayOption=signals
  mu_x_ash_f : Constant  Value=mu_x_ash_f
  mu_x_ash_r : Constant  Value=mu_x_ash_r
  mu_y_ash_f : Constant  Value=mu_y_ash_f
  mu_y_ash_r : Constant  Value=mu_y_ash_r
  Out1 : Outport  OutDataTypeStr=double  SampleTime=Ts
  wires:
  mu_x_ash_f/1 -> Mux/1  "mu_x_ash_f"
  mu_y_ash_f/1 -> Mux/2  "mu_y_ash_f"
  Cx_ash_f/1 -> Mux/3  "Cx_ash_f"
  Cy_ash_f/1 -> Mux/4  "Cy_ash_f"
  Bx_ash_f/1 -> Mux/5  "Bx_ash_f"
  By_ash_f/1 -> Mux/6  "By_ash_f"
  Ex_ash_f/1 -> Mux/7  "Ex_ash_f"
  Ey_ash_f/1 -> Mux/8  "E_y_ash_f"
  Cy_ash_r/1 -> Mux/12  "Cy_ash_r"
  Cx_ash_r/1 -> Mux/11  "Cx_ash_r"
  By_ash_r/1 -> Mux/14  "By_ash_r"
  Bx_ash_r/1 -> Mux/13  "Bx_ash_r"
  mu_y_ash_r/1 -> Mux/10  "mu_y_ash_r"
  Ex_ash_r/1 -> Mux/15  "Ex_ash_r"
  mu_x_ash_r/1 -> Mux/9  "mu_x_ash_r"
  Ey_ash_r/1 -> Mux/16  "Ey_ash_r"
  Mux/1 -> Out1/1

== system RajamaniController/control_model/3DoF_Vehicle/Subsystem1/Pacjeka_parameters_Subsystem/Ice_condition_subsystem ==
  Action Port : ActionPort  ActionType=case
  Bx_ice_f : Constant  Value=Bx_ash_f
  Bx_ice_r : Constant  Value=Bx_ash_r
  By_ice_f : Constant  Value=By_ash_f
  By_ice_r : Constant  Value=By_ash_r
  Cx_ice_f : Constant  Value=Cx_ash_f
  Cx_ice_r : Constant  Value=Cx_ash_r
  Cy_ice_f : Constant  Value=Cy_ash_f
  Cy_ice_r : Constant  Value=Cy_ash_r
  Ex_ice_f : Constant  Value=Ex_ash_f
  Ex_ice_r : Constant  Value=Ex_ash_r
  Ey_ice_f : Constant  Value=Ey_ash_f
  Ey_ice_r : Constant  Value=Ey_ash_r
  Mux : Mux  Inputs=16
      settings: DisplayOption=signals
  mu_x_ice_f : Constant  Value=mu_x_ash_f
  mu_x_ice_r : Constant  Value=mu_x_ash_r
  mu_y_ice_f : Constant  Value=mu_y_ash_f
  mu_y_ice_r : Constant  Value=mu_y_ash_r
  Out1 : Outport  OutDataTypeStr=double  SampleTime=Ts
  wires:
  mu_x_ice_f/1 -> Mux/1  "mu_x_ice_f"
  mu_y_ice_f/1 -> Mux/2  "mu_y_ice_f"
  Cx_ice_f/1 -> Mux/3  "Cx_ice_f"
  Cy_ice_f/1 -> Mux/4  "Cy_ice_f"
  Bx_ice_f/1 -> Mux/5  "Bx_ice_f"
  By_ice_f/1 -> Mux/6  "By_ice_f"
  Ex_ice_f/1 -> Mux/7  "Ex_ice_f"
  Ey_ice_f/1 -> Mux/8  "E_y_ice_f"
  Cy_ice_r/1 -> Mux/12  "Cy_ice_r"
  Cx_ice_r/1 -> Mux/11  "Cx_ice_r"
  By_ice_r/1 -> Mux/14  "By_ice_r"
  Bx_ice_r/1 -> Mux/13  "Bx_ice_r"
  mu_y_ice_r/1 -> Mux/10  "mu_y_ice_r"
  Ex_ice_r/1 -> Mux/15  "Ex_ice_r"
  mu_x_ice_r/1 -> Mux/9  "mu_x_ice_r"
  Ey_ice_r/1 -> Mux/16  "Ey_ice_r"
  Mux/1 -> Out1/1

== system RajamaniController/control_model/3DoF_Vehicle/Subsystem1/Pacjeka_parameters_Subsystem/Snow_condition_subsystem ==
  Action Port : ActionPort  ActionType=case
  Bx_snow_f : Constant  Value=Bx_snow_f
  Bx_snow_r : Constant  Value=Bx_snow_r
  By_snow_f : Constant  Value=By_snow_f
  By_snow_r : Constant  Value=By_snow_r
  Cx_snow_f : Constant  Value=Cx_snow_f
  Cx_snow_r : Constant  Value=Cx_snow_r
  Cy_snow_f : Constant  Value=Cy_snow_f
  Cy_snow_r : Constant  Value=Cy_snow_r
  Ex_snow_f : Constant  Value=Ex_snow_f
  Ex_snow_r : Constant  Value=Ex_snow_r
  Ey_snow_f : Constant  Value=Ey_snow_f
  Ey_snow_r : Constant  Value=Ey_snow_r
  Mux : Mux  Inputs=16
  mu_x_snow_f : Constant  Value=mu_x_snow_f
  mu_x_snow_r : Constant  Value=mu_x_snow_r
  mu_y_snow_f : Constant  Value=mu_y_snow_f
  mu_y_snow_r : Constant  Value=mu_y_snow_r
  Out1 : Outport  OutDataTypeStr=double  SampleTime=Ts
  wires:
  Ex_snow_r/1 -> Mux/15
  Cy_snow_r/1 -> Mux/12
  By_snow_r/1 -> Mux/14
  Cx_snow_r/1 -> Mux/11
  mu_y_snow_r/1 -> Mux/10
  mu_x_snow_r/1 -> Mux/9
  Bx_snow_r/1 -> Mux/13
  Ey_snow_r/1 -> Mux/16
  mu_x_snow_f/1 -> Mux/1
  mu_y_snow_f/1 -> Mux/2
  Cx_snow_f/1 -> Mux/3
  Cy_snow_f/1 -> Mux/4
  Bx_snow_f/1 -> Mux/5
  By_snow_f/1 -> Mux/6
  Ex_snow_f/1 -> Mux/7
  Ey_snow_f/1 -> Mux/8
  Mux/1 -> Out1/1

== system RajamaniController/control_model/3DoF_Vehicle/Subsystem1/Pacjeka_parameters_Subsystem/WetAshphalt_condition_subsystem ==
  Action Port : ActionPort  ActionType=case
  Bx_wash_f : Constant  Value=Bx_wash_f
  Bx_wash_r : Constant  Value=Bx_wash_r
  By_wash_f : Constant  Value=By_wash_f
  By_wash_r : Constant  Value=By_wash_r
  Cx_wash_f : Constant  Value=Cx_wash_f
  Cx_wash_r : Constant  Value=Cx_wash_r
  Cy_wash_f : Constant  Value=Cy_wash_f
  Cy_wash_r : Constant  Value=Cy_wash_r
  Ex_wash_f : Constant  Value=Ex_wash_f
  Ex_wash_r : Constant  Value=Ex_wash_r
  Ey_wash_f : Constant  Value=Ey_wash_f
  Ey_wash_r : Constant  Value=Ey_wash_r
  Mux : Mux  Inputs=16
      settings: DisplayOption=signals
  mu_x_wash_f : Constant  Value=mu_x_wash_f
  mu_x_wash_r : Constant  Value=mu_x_wash_r
  mu_y_wash_f : Constant  Value=mu_y_wash_f
  mu_y_wash_r : Constant  Value=mu_y_wash_r
  Out1 : Outport  OutDataTypeStr=double  SampleTime=Ts
  wires:
  mu_x_wash_f/1 -> Mux/1  "mu_x_wash_f"
  mu_y_wash_f/1 -> Mux/2  "mu_y_wash_f"
  Cx_wash_f/1 -> Mux/3  "Cx_wash_f"
  Cy_wash_f/1 -> Mux/4  "Cy_wash_f"
  Bx_wash_f/1 -> Mux/5  "Bx_wash_f"
  By_wash_f/1 -> Mux/6  "By_wash_f"
  Ex_wash_f/1 -> Mux/7  "Ex_wash_f"
  Ey_wash_f/1 -> Mux/8  "E_y_wash_f"
  Cy_wash_r/1 -> Mux/12  "Cy_wash_r"
  Cx_wash_r/1 -> Mux/11  "Cx_wash_r"
  By_wash_r/1 -> Mux/14  "By_wash_r"
  Bx_wash_r/1 -> Mux/13  "Bx_wash_r"
  mu_y_wash_r/1 -> Mux/10  "mu_y_wash_r"
  Ex_wash_r/1 -> Mux/15  "Ex_wash_r"
  mu_x_wash_r/1 -> Mux/9  "mu_x_wash_r"
  Ey_wash_r/1 -> Mux/16  "Ey_wash_r"
  Mux/1 -> Out1/1

== system RajamaniController/control_model/3DoF_Vehicle/Subsystem1/Vxdot_subsystem/Fy_subsystem ==
  Fyf : Inport
  Fxf : Inport  Port=2
  Fxr : Inport  Port=3
  cosDelta : Inport  Port=4
  sinDelta : Inport  Port=5
  Add : Sum  Inputs=-++
  Multiply : Product
  Multiply1 : Product
  Fx : Outport
  wires:
  Fyf/1 -> Multiply/1
  Multiply/1 -> Add/1
  Multiply1/1 -> Add/3
  Add/1 -> Fx/1
  Fxf/1 -> Multiply1/1
  cosDelta/1 -> Multiply1/2
  Fxr/1 -> Add/2
  sinDelta/1 -> Multiply/2

== system RajamaniController/control_model/3DoF_Vehicle/Subsystem1/Vydot_subsystem/Fy_subsystem ==
  Fyf : Inport
  Fyr : Inport  Port=2
  Fxf : Inport  Port=3
  cosDelta : Inport  Port=4
  sinDelta : Inport  Port=5
  Add : Sum  Inputs=3
  Multiply : Product
  Multiply1 : Product
  Fy : Outport
  wires:
  Fyf/1 -> Multiply/1
  cosDelta/1 -> Multiply/2
  Multiply/1 -> Add/1
  Fyr/1 -> Add/2
  Fxf/1 -> Multiply1/1
  sinDelta/1 -> Multiply1/2
  Multiply1/1 -> Add/3
  Add/1 -> Fy/1
